simulink model "dynamic_discrete_simulation_synth"  (R2020b)
settings: Solver=FixedStepAuto  StartTime=time_start  StopTime=time_end  FixedStep=dt  RelTol=1e-3
values from neighbouring files (symbols this model uses):
  B = 10    [hinfCostFunc.m]    (also in hinf_analysis_z.m; hinf_cmd_lmi.m = [zeros(4,2); Sigma.B]; init_rob_synth_sim.m; muCostFunc.m = 11)
  dt = 1e-3    (= 0.001)    [init_rob_synth_sim.m]    (also in read_data.m)
  dth0 = dq0    [init_rob_synth_sim.m]
  dv = 1e-3    (= 0.001)    [init_rob_synth_sim.m]
  Fc = Fs    [init_rob_synth_sim.m]
  Fs = [0.9, 1.3, 0.5]    [init_rob_synth_sim.m]
  Fv = diag([0.5,0.37,0.7])    [init_rob_synth_sim.m]
  K = 150    [hinfCostFunc.m]    (also in hinf_analysis_z.m; init_rob_synth_sim.m; muCostFunc.m = ureal('K',160,'Percentage',50); mu_analysis_z.m = ureal('K',160,'Percentage',50))
  Kj = [1;1;1]*5    [init_rob_synth_sim.m]
  Kjd = [1;1;1]*0.1    [init_rob_synth_sim.m]
  Kv = [2500;1500;2000]/256    [init_rob_synth_sim.m]
  Kvi = [3000;900;1000]/65536    [init_rob_synth_sim.m]
  M = 0.45    [hinfCostFunc.m]    (also in hinf_analysis_z.m; init_rob_synth_sim.m; muCostFunc.m = 0.42; mu_analysis_z.m = 0.42)
  nu = [0.8554, 0.5780, 0.9997]    [init_rob_synth_sim.m]
  R = [156;100;71]    [init_rob_synth_sim.m]
  tau_0 = [1.0000; 0.6119; 0.8268]    [init_rob_synth_sim.m]
  tau_m = 1/(10*2*pi)    (= 0.0159154943092)    [hinfCostFunc.m]    (also in hinf_analysis_z.m; init_rob_synth_sim.m; muCostFunc.m; mu_analysis_z.m)
  Tc = [0.0335;0.0335;0.051]    [init_rob_synth_sim.m]
  th0 = theta_DH(2:4) - (q0 - KUKA_offset(2:4))    [init_rob_synth_sim.m]
  thmax = theta_DH - (qmin - KUKA_offset)    [init_rob_synth_sim.m]
  thmin = theta_DH - (qmax - KUKA_offset)    [init_rob_synth_sim.m]
undefined symbols (not defined in the file or in its folder): den_W1, den_W2, den_W3, num_W1, num_W2, num_W3
libraries: simulink x1
settings Model: Creator=fortineau_vin  LastModifiedBy=fortineau_vin
settings DataIOCC: ReturnWorkspaceOutputs=off
settings DebuggingCC: ArithmeticOperatorsInVariantConditions=warning
settings SFSimCC: SimUseLocalCustomCode=off  CustomCodeUndefinedFunction=UseInterfaceOnly
settings RTWCC: RTWUseLocalCustomCode=off

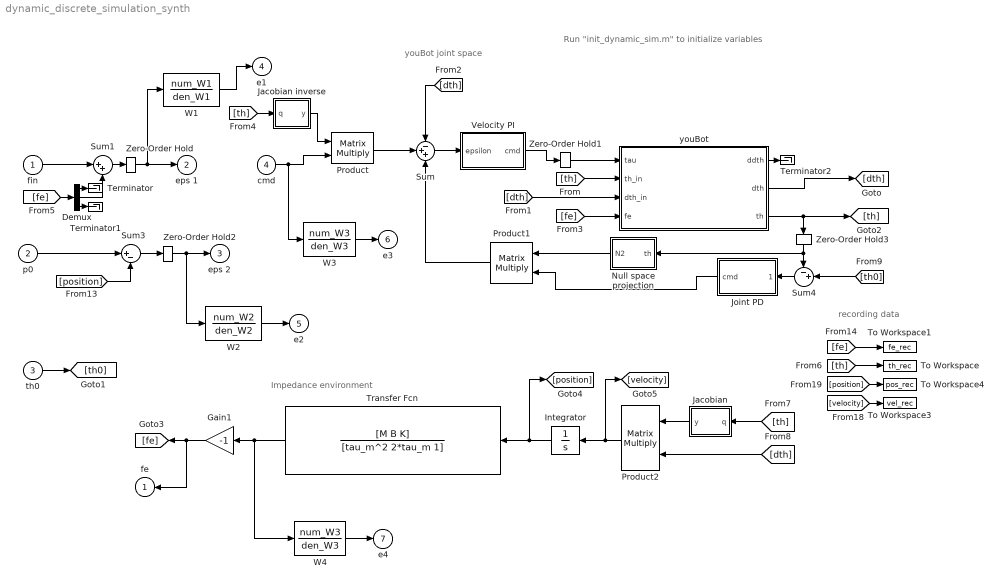
== system dynamic_discrete_simulation_synth ==
  note: recording data
  note: Run "init_dynamic_sim.m" to initialize variables
  note: youBot joint space
  note: Impedance environment
  fin : Inport
  p0 : Inport  Port=2
  th0 : Inport  Port=3
  cmd : Inport  Port=4
  Demux : Demux  Outputs=3
  Gain1 : Gain  Gain=-1
  Integrator : Integrator
  Jacobian : MATLAB Function  TreatAsAtomicUnit=on
  Jacobian inverse : MATLAB Function  TreatAsAtomicUnit=on
  Joint PD : Subsystem
  Null space projection : Subsystem
  Product : Product  Multiplication=Matrix(*)
  Product1 : Product  Multiplication=Matrix(*)
  Product2 : Product  Multiplication=Matrix(*)
  Sum : Sum  Inputs=-++
  Sum1 : Sum  Inputs=|++
  Sum3 : Sum  Inputs=|+-
  Sum4 : Sum  Inputs=-+|
  Terminator : Terminator
  Terminator1 : Terminator
  Terminator2 : Terminator
  To Workspace : ToWorkspace  VariableName=th_rec  SaveFormat=Structure  SampleTime=1e-3
      settings: Save2DSignal=2-D array (concatenate along first dimension)
  To Workspace1 : ToWorkspace  VariableName=fe_rec  SaveFormat=Structure  SampleTime=1e-3
      settings: Save2DSignal=2-D array (concatenate along first dimension)
  To Workspace3 : ToWorkspace  VariableName=vel_rec  SaveFormat=Structure  SampleTime=1e-3
      settings: Save2DSignal=2-D array (concatenate along first dimension)
  To Workspace4 : ToWorkspace  VariableName=pos_rec  SaveFormat=Structure  SampleTime=1e-3
      settings: Save2DSignal=2-D array (concatenate along first dimension)
  Transfer Fcn : TransferFcn  Numerator=[M B K]  Denominator=[tau_m^2 2*tau_m 1]
  Velocity PI : Subsystem
  W1 : TransferFcn  Numerator=num_W1  Denominator=den_W1
  W2 : TransferFcn  Numerator=num_W2  Denominator=den_W2
  W3 : TransferFcn  Numerator=num_W3  Denominator=den_W3
  W4 : TransferFcn  Numerator=num_W3  Denominator=den_W3
  Zero-Order Hold{,1..3} (4 alike) : ZeroOrderHold  SampleTime=dt
  youBot : Subsystem
  fe : Outport
  eps 1 : Outport  Port=2
  eps 2 : Outport  Port=3
  e1 : Outport  Port=4
  e2 : Outport  Port=5
  e3 : Outport  Port=6
  e4 : Outport  Port=7
  wires:
  Velocity PI/1(cmd) -> Zero-Order Hold1/1
  Sum/1 -> Velocity PI/1(epsilon)
  [dth] -> Sum/1
  Product/1 -> Sum/2
  Sum1/1 -> Zero-Order Hold/1
  [th] -> Jacobian inverse/1(q)
  Sum3/1 -> Zero-Order Hold2/1
  p0/1 -> Sum3/1
  [position] -> Sum3/2
  [th] -> To Workspace/1
  [fe] -> To Workspace1/1
  [th] -> youBot/2(th_in)
  [dth] -> youBot/3(dth_in)
  youBot/1(ddth) -> Terminator2/1
  youBot/2(dth) -> [dth]
  Sum4/1 -> Joint PD/1(epsilon)
  [th0] -> Sum4/2
  Null space projection/1(N2) -> Product1/1
  youBot/3(th) -> [th], Zero-Order Hold3/1
  Joint PD/1(cmd) -> Product1/2
  Product1/1 -> Sum/3
  [velocity] -> To Workspace3/1
  [position] -> To Workspace4/1
  cmd/1 -> W3/1, Product/2
  Jacobian inverse/1(y) -> Product/1
  Demux/2 -> Sum1/2
  Zero-Order Hold1/1 -> youBot/1(tau)
  [fe] -> Demux/1
  [fe] -> youBot/4(fe)
  Demux/1 -> Terminator/1
  Demux/3 -> Terminator1/1
  Zero-Order Hold/1 -> eps 1/1, W1/1
  Zero-Order Hold2/1 -> W2/1, eps 2/1
  Zero-Order Hold3/1 -> Null space projection/1(th), Sum4/1
  fin/1 -> Sum1/1
  [th] -> Jacobian/1(q)
  [dth] -> Product2/2
  Jacobian/1(y) -> Product2/1
  th0/1 -> [th0]
  Gain1/1 -> fe/1, [fe]
  Transfer Fcn/1 -> W4/1, Gain1/1
  Integrator/1 -> [position], Transfer Fcn/1
  Product2/1 -> [velocity], Integrator/1
  W1/1 -> e1/1
  W2/1 -> e2/1
  W3/1 -> e3/1
  W4/1 -> e4/1

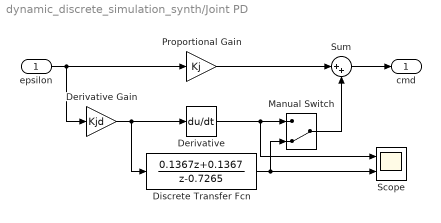
== system dynamic_discrete_simulation_synth/Joint PD ==
  epsilon : Inport
  " Derivative Gain" : Gain  Gain=Kjd
  Derivative : Derivative
  Discrete Transfer Fcn : DiscreteTransferFcn  Numerator=[0.1367 0.1367]  Denominator=[1 -0.7265]
  Manual Switch : ManualSwitch  CurrentSetting=0
  Proportional Gain : Gain  Gain=Kj
  Scope : Scope  NumInputPorts=2
  Sum : Sum  Inputs=|++
  cmd : Outport  VectorParamsAs1DForOutWhenUnconnected=off
  wires:
  Sum/1 -> cmd/1
  epsilon/1 -> " Derivative Gain"/1, Proportional Gain/1
  " Derivative Gain"/1 -> Derivative/1, Discrete Transfer Fcn/1
  Proportional Gain/1 -> Sum/1
  Derivative/1 -> Scope/1, Manual Switch/1
  Manual Switch/1 -> Sum/2
  Discrete Transfer Fcn/1 -> Scope/2, Manual Switch/2

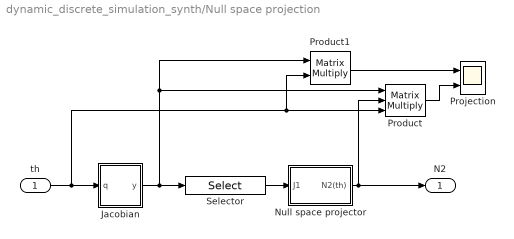
== system dynamic_discrete_simulation_synth/Null space projection ==
  th : Inport
  Jacobian : MATLAB Function  TreatAsAtomicUnit=on
  Null space projector : Subsystem
  Product : Product  Inputs=3  Multiplication=Matrix(*)
  Product1 : Product  Multiplication=Matrix(*)
  Projection : Scope  NumInputPorts=2
  Selector : Selector  NumberOfDimensions=2  InputPortWidth=3  IndexOptions=Index vector (dialog),Index vector (dialog)  Indices=2,[1 2 3]  OutputSizes=1,1
  N2 : Outport  VectorParamsAs1DForOutWhenUnconnected=off
  wires:
  Null space projector/1(N2(th)) -> N2/1, Product/2
  Jacobian/1(y) -> Product1/1, Product/1, Selector/1
  Selector/1 -> Null space projector/1(J1)
  th/1 -> Product1/2, Product/3, Jacobian/1(q)
  Product/1 -> Projection/2
  Product1/1 -> Projection/1

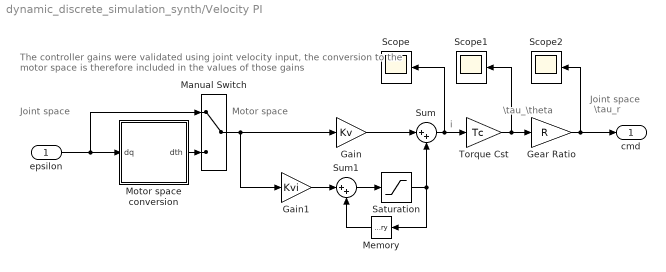
== system dynamic_discrete_simulation_synth/Velocity PI ==
  note: The controller gains were validated using joint velocity input, the conversion to
      | the motor space is therefore included in the values of those gains
  note: \tau_\theta
  note: i
  note: Motor space
  note: Joint space
  note: \tau_r
  note: Joint space
  epsilon : Inport
  Gain : Gain  Gain=Kv
  Gain1 : Gain  Gain=Kvi
  Gear Ratio : Gain  Gain=R
  Manual Switch : ManualSwitch
  Memory : Memory
  Motor space conversion : Subsystem
  Saturation : Saturate  UpperLimit=100  LowerLimit=-100
  Scope : Scope
  Scope1 : Scope
  Scope2 : Scope
  Sum : Sum  Inputs=|++
  Sum1 : Sum  Inputs=|++
  Torque Cst : Gain  Gain=Tc
  cmd : Outport  VectorParamsAs1DForOutWhenUnconnected=off
  wires:
  Gain/1 -> Sum/1
  Saturation/1 -> Sum/2, Memory/1
  Gear Ratio/1 -> Scope2/1, cmd/1
  Sum/1 -> Scope/1, Torque Cst/1
  Torque Cst/1 -> Scope1/1, Gear Ratio/1
  epsilon/1 -> Manual Switch/1, Motor space conversion/1(dq)
  Motor space conversion/1(dth) -> Manual Switch/2
  Manual Switch/1 -> Gain/1, Gain1/1
  Sum1/1 -> Saturation/1
  Memory/1 -> Sum1/2
  Gain1/1 -> Sum1/1

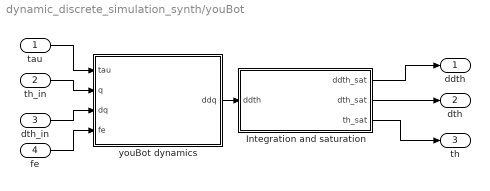
== system dynamic_discrete_simulation_synth/youBot ==
  tau : Inport
  th_in : Inport  Port=2
  dth_in : Inport  Port=3
  fe : Inport  Port=4
  Integration and saturation : Subsystem
  youBot dynamics : Subsystem
  ddth : Outport  VectorParamsAs1DForOutWhenUnconnected=off
  dth : Outport  Port=2  VectorParamsAs1DForOutWhenUnconnected=off
  th : Outport  Port=3  VectorParamsAs1DForOutWhenUnconnected=off
  wires:
  tau/1 -> youBot dynamics/1(tau)
  youBot dynamics/1(ddq) -> Integration and saturation/1(ddth)
  dth_in/1 -> youBot dynamics/3("dq ")
  th_in/1 -> youBot dynamics/2("q ")
  fe/1 -> youBot dynamics/4(fe)
  Integration and saturation/3(th_sat) -> th/1
  Integration and saturation/1(ddth_sat) -> ddth/1
  Integration and saturation/2(dth_sat) -> dth/1

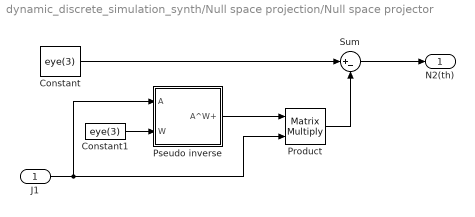
== system dynamic_discrete_simulation_synth/Null space projection/Null space projector ==
  J1 : Inport
  Constant : Constant  Value=eye(3)  VectorParams1D=off
  Constant1 : Constant  Value=eye(3)  VectorParams1D=off
  Product : Product  Multiplication=Matrix(*)
  Pseudo inverse : Subsystem
  Sum : Sum  Inputs=|+-
  N2(th) : Outport  VectorParamsAs1DForOutWhenUnconnected=off
  wires:
  Constant/1 -> Sum/1
  Constant1/1 -> Pseudo inverse/2(W)
  J1/1 -> Pseudo inverse/1(A), Product/2
  Pseudo inverse/1(A^W+) -> Product/1
  Product/1 -> Sum/2
  Sum/1 -> N2(th)/1

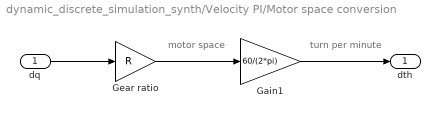
== system dynamic_discrete_simulation_synth/Velocity PI/Motor space conversion ==
  note: motor space
  note: turn per minute
  dq : Inport
  Gain1 : Gain  Gain=60/(2*pi)
  Gear ratio : Gain  Gain=R
  dth : Outport  VectorParamsAs1DForOutWhenUnconnected=off
  wires:
  dq/1 -> Gear ratio/1
  Gear ratio/1 -> Gain1/1
  Gain1/1 -> dth/1

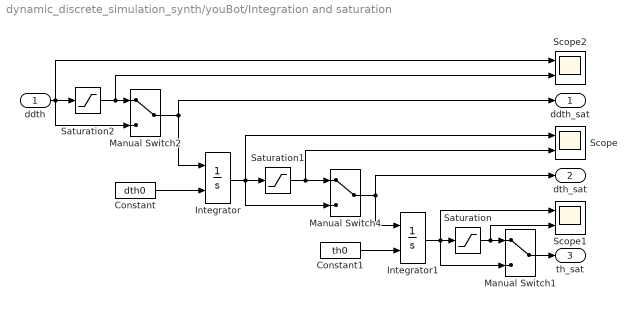
== system dynamic_discrete_simulation_synth/youBot/Integration and saturation ==
  ddth : Inport
  Constant : Constant  Value=dth0
  Constant1 : Constant  Value=th0
  Integrator : Integrator  InitialConditionSource=external
  Integrator1 : Integrator  InitialConditionSource=external
  Manual Switch1 : ManualSwitch
  Manual Switch2 : ManualSwitch
  Manual Switch4 : ManualSwitch
  Saturation : Saturate  UpperLimit=thmax(2:4)'  LowerLimit=thmin(2:4)'
  Saturation1 : Saturate  UpperLimit=[2.685122; 4.188790; 5.899705]  LowerLimit=[-2.685122; -4.188790; -5.899705]
  Saturation2 : Saturate  UpperLimit=[10;10;10]  LowerLimit=[-10;-10;-10]
  Scope : Scope  NumInputPorts=2
  Scope1 : Scope  NumInputPorts=2
  Scope2 : Scope  NumInputPorts=2
  ddth_sat : Outport  VectorParamsAs1DForOutWhenUnconnected=off
  dth_sat : Outport  Port=2  VectorParamsAs1DForOutWhenUnconnected=off
  th_sat : Outport  Port=3  VectorParamsAs1DForOutWhenUnconnected=off
  wires:
  Manual Switch2/1 -> ddth_sat/1, Integrator/1
  Manual Switch1/1 -> th_sat/1
  Manual Switch4/1 -> Integrator1/1, dth_sat/1
  ddth/1 -> Scope2/1, Manual Switch2/2, Saturation2/1
  Saturation2/1 -> Scope2/2, Manual Switch2/1
  Saturation1/1 -> Scope/2, Manual Switch4/1
  Saturation/1 -> Scope1/2, Manual Switch1/1
  Constant/1 -> Integrator/2
  Integrator/1 -> Scope/1, Manual Switch4/2, Saturation1/1
  Integrator1/1 -> Scope1/1, Manual Switch1/2, Saturation/1
  Constant1/1 -> Integrator1/2

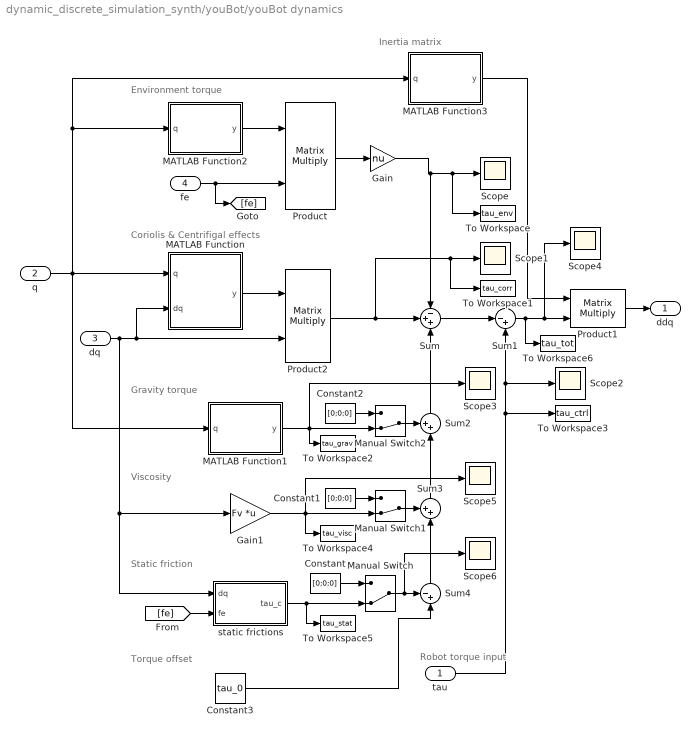
== system dynamic_discrete_simulation_synth/youBot/youBot dynamics ==
  note: Coriolis & Centrifigal effects
  note: Gravity torque
  note: Environment torque
  note: Robot torque input
  note: Inertia matrix
  note: Viscosity
  note: Static friction
  note: Torque offset
  tau : Inport
  "q " : Inport  Port=2
  "dq " : Inport  Port=3
  fe : Inport  Port=4
  Constant : Constant  Value=[0;0;0]
  Constant1 : Constant  Value=[0;0;0]
  Constant2 : Constant  Value=[0;0;0]
  Constant3 : Constant  Value=tau_0
  Gain : Gain  Gain=nu
  Gain1 : Gain  Gain=Fv  Multiplication=Matrix(K*u)
  MATLAB Function : MATLAB Function  TreatAsAtomicUnit=on
  MATLAB Function1 : MATLAB Function  TreatAsAtomicUnit=on
  MATLAB Function2 : MATLAB Function  TreatAsAtomicUnit=on
  MATLAB Function3 : MATLAB Function  TreatAsAtomicUnit=on
  Manual Switch : ManualSwitch  CurrentSetting=0
  Manual Switch1 : ManualSwitch  CurrentSetting=0
  Manual Switch2 : ManualSwitch  CurrentSetting=0
  Product : Product  Multiplication=Matrix(*)
  Product1 : Product  Multiplication=Matrix(*)
  Product2 : Product  Multiplication=Matrix(*)
  Scope{,1..6} (7 alike) : Scope
  Sum : Sum  Inputs=-++
  Sum1 : Sum  Inputs=|-+
  Sum2 : Sum  Inputs=++|
  Sum3 : Sum  Inputs=++|
  Sum4 : Sum  Inputs=-+|
  To Workspace : ToWorkspace  VariableName=tau_env  SaveFormat=Timeseries  SampleTime=-1
  To Workspace1 : ToWorkspace  VariableName=tau_corr  SaveFormat=Timeseries  SampleTime=-1
  To Workspace2 : ToWorkspace  VariableName=tau_grav  SaveFormat=Timeseries  SampleTime=-1
  To Workspace3 : ToWorkspace  VariableName=tau_ctrl  SaveFormat=Timeseries  SampleTime=-1
  To Workspace4 : ToWorkspace  VariableName=tau_visc  SaveFormat=Timeseries  SampleTime=-1
  To Workspace5 : ToWorkspace  VariableName=tau_stat  SaveFormat=Timeseries  SampleTime=-1
  To Workspace6 : ToWorkspace  VariableName=tau_tot  SaveFormat=Timeseries  SampleTime=-1
  static frictions : Subsystem
  ddq : Outport  VectorParamsAs1DForOutWhenUnconnected=off
  wires:
  "dq "/1 -> Product2/2, MATLAB Function/2(dq), static frictions/1(dq), Gain1/1
  "q "/1 -> MATLAB Function/1(q), MATLAB Function2/1(q), MATLAB Function3/1(q), MATLAB Function1/1(q)
  Product/1 -> Gain/1
  Product1/1 -> ddq/1
  MATLAB Function1/1(y) -> Scope3/1, Manual Switch2/2, To Workspace2/1
  Sum/1 -> Sum1/1
  Product2/1 -> Scope1/1, To Workspace1/1, Sum/2
  MATLAB Function/1(y) -> Product2/1
  MATLAB Function2/1(y) -> Product/1
  fe/1 -> Product/2, [fe]
  MATLAB Function3/1(y) -> Product1/1
  Sum1/1 -> To Workspace6/1, Scope4/1, Product1/2
  tau/1 -> To Workspace3/1, Scope2/1, Sum1/2
  Gain/1 -> Scope/1, To Workspace/1, Sum/1
  Sum2/1 -> Sum/3
  Gain1/1 -> Manual Switch1/2, Scope5/1, To Workspace4/1
  [fe] -> static frictions/2(fe)
  Sum3/1 -> Sum2/2
  static frictions/1(tau_c) -> To Workspace5/1, Manual Switch/2
  Constant/1 -> Manual Switch/1
  Constant1/1 -> Manual Switch1/1
  Manual Switch1/1 -> Sum3/1
  Manual Switch2/1 -> Sum2/1
  Constant2/1 -> Manual Switch2/1
  Sum4/1 -> Sum3/2
  Manual Switch/1 -> Scope6/1, Sum4/1
  Constant3/1 -> Sum4/2

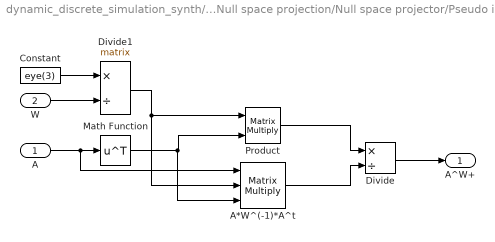
== system dynamic_discrete_simulation_synth/Null space projection/Null space projector/Pseudo inverse ==
  A : Inport
  W : Inport  Port=2
  A*W^(-1)*A^t : Product  Inputs=3  Multiplication=Matrix(*)
  Constant : Constant  Value=eye(3)
  Divide : Product  Inputs=*/
  Divide1 : Product  Inputs=*/  Multiplication=Matrix(*)
  Math Function : Math  Operator=transpose  SignedPower=on  SaturateOnIntegerOverflow=on
  Product : Product  Multiplication=Matrix(*)
  A^W+ : Outport  VectorParamsAs1DForOutWhenUnconnected=off
  wires:
  W/1 -> Divide1/2
  A/1 -> A*W^(-1)*A^t/1, Math Function/1
  Math Function/1 -> A*W^(-1)*A^t/3, Product/2
  Divide1/1 -> A*W^(-1)*A^t/2, Product/1
  Product/1 -> Divide/1
  A*W^(-1)*A^t/1 -> Divide/2
  Divide/1 -> A^W+/1
  Constant/1 -> Divide1/1

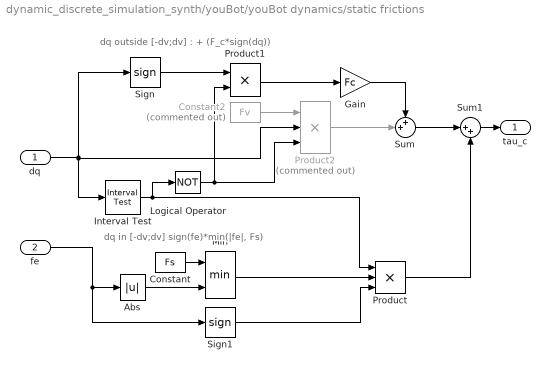
== system dynamic_discrete_simulation_synth/youBot/youBot dynamics/static frictions ==
  note: dq in [-dv;dv]
      |
      | sign(fe)*min(|fe|, Fs)
  note: dq outside [-dv;dv] : + (F_c*sign(dq))
  dq : Inport
  fe : Inport  Port=2
  Abs : Abs
  Constant : Constant  Value=Fs
  Constant2 : Constant  Commented=on  Value=Fv
  Gain : Gain  Gain=Fc
  Interval Test : simulink/Logic and Bit Operations/Interval Test  IntervalClosedRight=on  uplimit=dv  IntervalClosedLeft=on  lowlimit=-dv  OutDataTypeStr=boolean
  Logical Operator : Logic  Operator=NOT  AllPortsSameDT=off  OutDataTypeStr=boolean
  Min : MinMax  Inputs=2
  Product : Product  Inputs=3
  Product1 : Product
  Product2 : Product  Commented=on  Inputs=3
  Sign : Signum
  Sign1 : Signum
  Sum : Sum  Inputs=++|
  Sum1 : Sum  Inputs=|++
  tau_c : Outport  VectorParamsAs1DForOutWhenUnconnected=off
  wires:
  Sum1/1 -> tau_c/1
  Interval Test/1 -> Logical Operator/1, Product/1
  fe/1 -> Sign1/1, Abs/1
  Abs/1 -> Min/2
  Constant/1 -> Min/1
  Min/1 -> Product/2
  Sign1/1 -> Product/3
  Logical Operator/1 -> Product1/2, Product2/3
  dq/1 -> Sign/1, Product2/2, Interval Test/1
  Constant2/1 -> Product2/1
  Product2/1 -> Sum/2
  Product1/1 -> Gain/1
  Sum/1 -> Sum1/1
  Product/1 -> Sum1/2
  Sign/1 -> Product1/1
  Gain/1 -> Sum/1

== matlab function dynamic_discrete_simulation_synth/youBot/youBot dynamics/MATLAB Function ==
  data: q input; y output; dq input
function y = C_sim(q,dq)
q2 = q(2);
q3 = q(3);
dq1 = dq(1);
dq2 = dq(2);
dq3 = dq(3);
y = C_3DOF(dq1,dq2,dq3,q2,q3);

== matlab function dynamic_discrete_simulation_synth/youBot/youBot dynamics/MATLAB Function2 ==
  data: q input; y output
function y = tJ_sim(q)
q1 = q(1);
q2 = q(2);
q3 = q(3);
y = J0E_3DOF(q1,q2,q3)';

== matlab function dynamic_discrete_simulation_synth/youBot/youBot dynamics/MATLAB Function3 ==
  data: q input; y output
function y = iM_sim(q)
q2 = q(2);
q3 = q(3);
y = iM_3DOF(q2,q3);

== matlab function dynamic_discrete_simulation_synth/Jacobian inverse ==
  data: q input; y output
function y = iJ(q)
q1 = q(1);
q2 = q(2);
q3 = q(3);
y = iJ0E_3DOF(q1,q2,q3);

== matlab function dynamic_discrete_simulation_synth/Null space projection/Jacobian ==
  data: q input; y output
function y = J(q)
q1 = q(1);
q2 = q(2);
q3 = q(3);
y = J0E_3DOF(q1,q2,q3);

== matlab function dynamic_discrete_simulation_synth/Jacobian ==
  data: q input; y output
function y = J(q)
q1 = q(1);
q2 = q(2);
q3 = q(3);
y = J0E_3DOF(q1,q2,q3);

== matlab function dynamic_discrete_simulation_synth/youBot/youBot dynamics/MATLAB Function1 ==
  data: q input; y output
function y = G_sim(q)
q1 = q(1);
q2 = q(2);
q3 = q(3);
y = G_3DOF(q1,q2,q3);
